simulink model "ultrasonic"  (R2022b)
settings: Solver=FixedStepDiscrete  StartTime=0.0  StopTime=10.0  FixedStep=1e-3  RelTol=1e-3  EnableMultiTasking=on
libraries: arduinolib x4, arduinosensorlib x1
settings Model: ExtModeTrigDuration=2  Creator=brbar  LastModifiedBy=brbar
settings OptimizationCC: EnhancedBackFolding=on  PassReuseOutputArgsAs=Individual arguments  ZeroExternalMemoryAtStartup=off  ZeroInternalMemoryAtStartup=off  MaxStackSize=64  OptimizeBlockOrder=speed  DifferentSizesBufferReuse=on  OptimizationCustomize=off  EfficientTunableParamExpr=on
settings DebuggingCC: ParameterTunabilityLossMsg=error
settings HardwareCC: ProdBitPerInt=16  ProdBitPerPointer=16  ProdBitPerSizeT=16  ProdBitPerPtrDiffT=16  ProdLargestAtomicFloat=None  ProdWordSize=8  ProdHWDeviceType=Atmel->AVR
settings SFSimCC: MATLABDynamicMemAlloc=off
settings RTWCC: Description=Embedded Coder  SystemTargetFile=ert.tlc  HardwareBoard=Arduino Uno  TLCOptions=-aInlineSetEventsForThisBaseRateFcn=TLC_FALSE -aSuppressMultiTaskScheduler=TLC_FALSE -aRateBasedStepFcn=1  TemplateMakefile=ert_default_tmf  Toolchain=Arduino AVR  BuildConfiguration=Faster Runs
settings CodeAppCC: ForceParamTrailComments=on  IgnoreCustomStorageClasses=off  OperatorAnnotations=on  SimulinkDataObjDesc=on  SFDataObjDesc=on  InsertBlockDesc=on
settings ERTTargetCC: SupportContinuousTime=on  SupportVariableSizeSignals=on  ExtModeTransport=3  ExtModeStaticAlloc=on  ExtModeAutomaticAllocSize=off  ExtModeStaticAllocSize=250  ExtModeMexFile=ext_xcp  ExtModeIntrfLevel=Level2 - Open

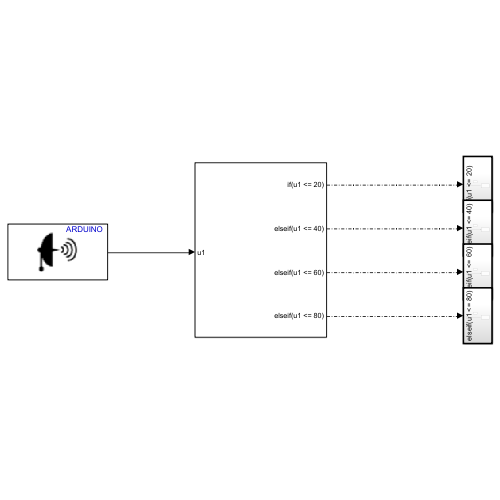
[thumbnail: Simulink's stored preview of the top-level diagram]
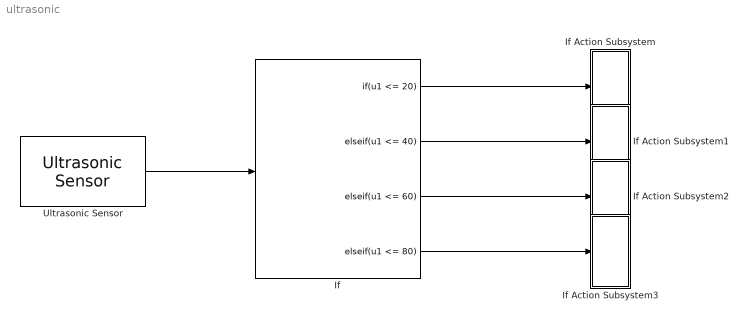
== system ultrasonic ==
  If : If  IfExpression=u1 <= 20  ElseIfExpressions=u1 <= 40,u1 <= 60,u1 <= 80  ShowElse=off
  If Action Subsystem : Subsystem  TreatAsAtomicUnit=on
  If Action Subsystem1 : Subsystem  TreatAsAtomicUnit=on
  If Action Subsystem2 : Subsystem  TreatAsAtomicUnit=on
  If Action Subsystem3 : Subsystem  TreatAsAtomicUnit=on
  Ultrasonic Sensor : arduinosensorlib/Ultrasonic Sensor  NumSignalPins=1  TrigPin=4  EchoPin=5  SignalPin=3  SampleTime_=0.1  blockPlatform=ARDUINO
  wires:
  If/1 -> If Action Subsystem/Action
  If/2 -> If Action Subsystem1/Action
  If/3 -> If Action Subsystem2/Action
  If/4 -> If Action Subsystem3/Action
  Ultrasonic Sensor/1 -> If/1

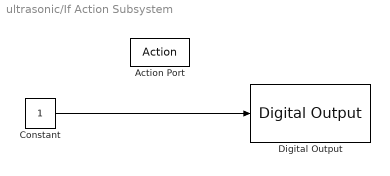
== system ultrasonic/If Action Subsystem ==
  Action Port : ActionPort  ActionPortLabel=if(u1 <= 20)
  Constant : Constant
  Digital Output : arduinolib/Digital Output  pinNumber=9  Direction=output  blockPlatform=arduino
  wires:
  Constant/1 -> Digital Output/1

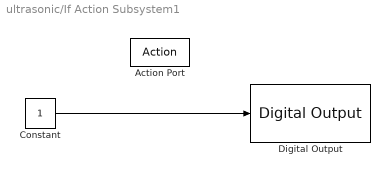
== system ultrasonic/If Action Subsystem1 ==
  Action Port : ActionPort  ActionPortLabel=elseif(u1 <= 40)
  Constant : Constant
  Digital Output : arduinolib/Digital Output  pinNumber=10  Direction=output  blockPlatform=arduino
  wires:
  Constant/1 -> Digital Output/1

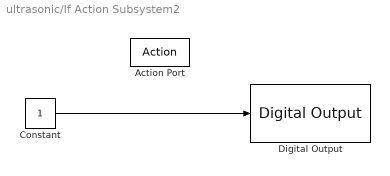
== system ultrasonic/If Action Subsystem2 ==
  Action Port : ActionPort  ActionPortLabel=elseif(u1 <= 60)
  Constant : Constant
  Digital Output : arduinolib/Digital Output  pinNumber=11  Direction=output  blockPlatform=arduino
  wires:
  Constant/1 -> Digital Output/1

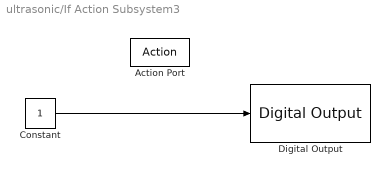
== system ultrasonic/If Action Subsystem3 ==
  Action Port : ActionPort  ActionPortLabel=elseif(u1 <= 80)
  Constant : Constant
  Digital Output : arduinolib/Digital Output  pinNumber=12  Direction=output  blockPlatform=arduino
  wires:
  Constant/1 -> Digital Output/1
